simulink model "HybridSkyGroundHookController"  (R2025b)
settings: Solver=VariableStepAuto  StartTime=0.0  StopTime=3  RelTol=1e-3
values from neighbouring files (symbols this model uses):
  cs = 1500    [RegenVariables.mat]
  Cskymax = 1500    [RegenVariables.mat]
  Cskymin = 0    [RegenVariables.mat]
  ks = 18000    [RegenVariables.mat]
  kt = 200000    [RegenVariables.mat]
  ms = 320    [RegenVariables.mat]
  mu = 45    [RegenVariables.mat]
settings Model: Creator=khalidwaleed  LastModifiedBy=khalidwaleed

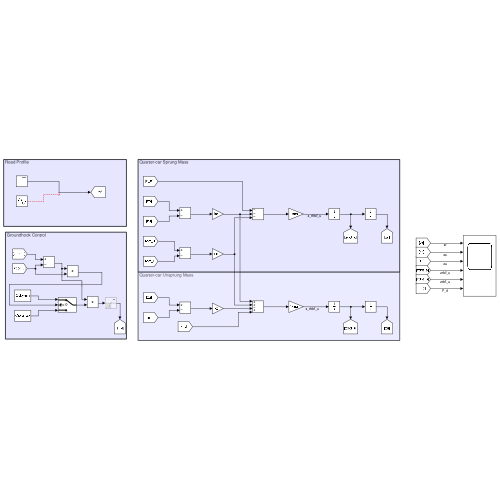
[thumbnail: Simulink's stored preview of the top-level diagram]
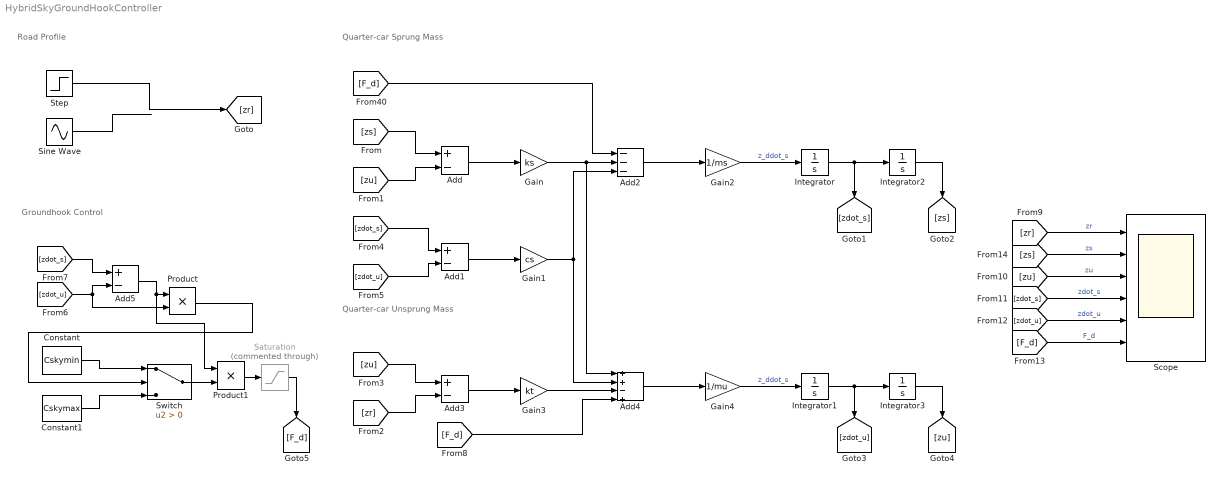
== system HybridSkyGroundHookController ==
  note: Road Profile
  note: Groundhook Control
  note: Quarter-car Sprung Mass
  note: Quarter-car Unsprung Mass
  Add{,1,3,5} (4 alike) : Sum  Inputs=+-
  Add2 : Sum  Inputs=---
  Add4 : Sum  Inputs=++-+
  Constant : Constant  Value=Cskymin
  Constant1 : Constant  Value=Cskymax
  Gain : Gain  Gain=ks
  Gain1 : Gain  Gain=cs
  Gain2 : Gain  Gain=1/ms
  Gain3 : Gain  Gain=kt
  Gain4 : Gain  Gain=1/mu
  Integrator{,1..3} (4 alike) : Integrator
  Product : Product
  Product1 : Product
  Saturation : Saturate  Commented=through  UpperLimit=2000  LowerLimit=-200
  Scope : Scope  NumInputPorts=6
      settings: ActiveDisplayString=6  ActiveDisplayYMinimum=-5745.5244927949361  ActiveDisplayYMaximum=2962.5003687134581
  Sine Wave : Sin  Amplitude=0.02  Frequency=10  SampleTime=0
  Step : Step  After=0.1  SampleTime=0
  Switch : Switch  Criteria=u2 > Threshold  ZeroCross=off  SaturateOnIntegerOverflow=off  InputSameDT=off
  wires:
  Gain2/1 -> Integrator/1  "z_ddot_s"
  [zr] -> Add3/2
  Integrator/1 -> Integrator2/1, [zdot_s]
  [zs] -> Add/1
  Add/1 -> Gain/1
  Integrator2/1 -> [zs]
  Integrator1/1 -> Integrator3/1, [zdot_u]
  [zdot_s] -> Add1/1
  Gain4/1 -> Integrator1/1  "z_ddot_s"
  Gain1/1 -> Add4/2, Add2/3
  Add2/1 -> Gain2/1
  [zu] -> Add3/1
  Add1/1 -> Gain1/1
  Gain3/1 -> Add4/3
  [zdot_u] -> Add1/2
  Add4/1 -> Gain4/1
  [F_d] -> Add2/1
  Integrator3/1 -> [zu]
  Gain/1 -> Add4/1, Add2/2
  [zu] -> Add/2
  Add3/1 -> Gain3/1
  Add5/1 -> Product1/1, Product/1
  [zdot_u] -> Product/2, Add5/2
  [zdot_s] -> Add5/1
  Product/1 -> Switch/2
  Constant/1 -> Switch/1
  Constant1/1 -> Switch/3
  Switch/1 -> Product1/2
  Step/1 -> [zr]
  Sine Wave/1 -> ?
  [F_d] -> Add4/4
  [zr] -> Scope/1  "zr"
  [F_d] -> Scope/6  "F_d"
  [zdot_u] -> Scope/5  "zdot_u"
  [zdot_s] -> Scope/4  "zdot_s"
  [zs] -> Scope/2  "zs"
  [zu] -> Scope/3  "zu"
  Product1/1 -> Saturation/1
  Saturation/1 -> [F_d]
